simulink model "fft_HIL"  (Simulink 7.0)
settings: Solver=FixedStepDiscrete  StartTime=0.0  StopTime=800  RelTol=1e-3
InitFcn:
  | %% DSPBuilder Start
  | alt_dspbuilder_update_model(bdroot)
  | %% DSPBuilder End
libraries: allblocks_alteradspbuilder2 x18, dspsrcs4 x4, simulink x3
settings Model: Creator=lkong  LastModifiedBy=lkong
settings OptimizationCC: InlineInvariantSignals=on
settings DebuggingCC: SaveWithParameterizedLinksMsg=none  SignalResolutionControl=TryResolveAllWithWarning  SolverPrmCheckMsg=none  MultiTaskDSMMsg=warning  MultiTaskCondExecSysMsg=none
settings HardwareCC: TargetUnknown=on
settings RTWCC: IncludeERTFirstTime=on
settings GRTTargetCC: TargetFcnLib=ansi_tfl_tmw.mat

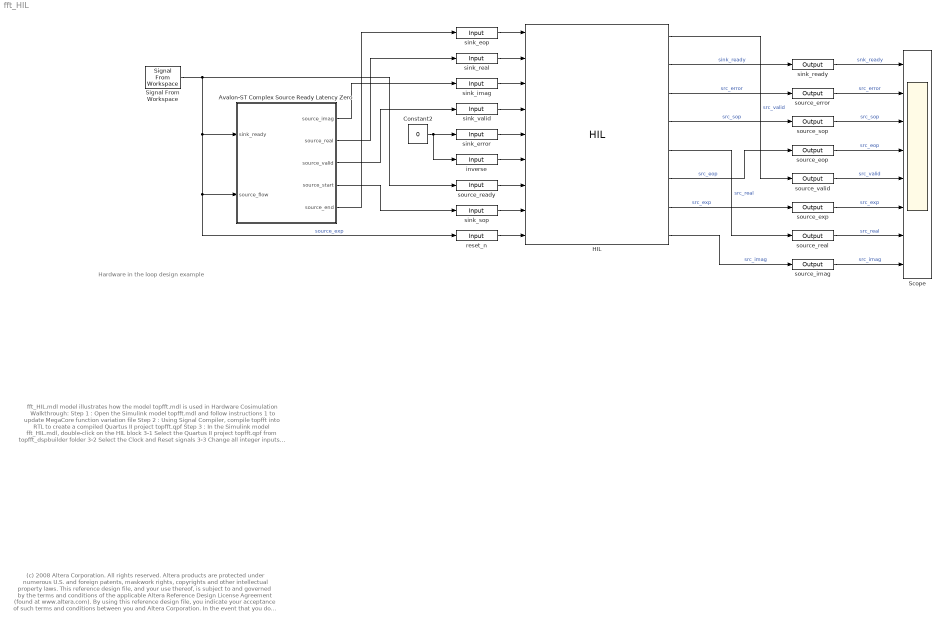
== system fft_HIL ==
  note: (c) 2008 Altera Corporation. All rights reserved.  Altera products are protected under numerous U.S. and foreign patents, maskwork rights, copyrights and other intellectual property laws.
      | This reference design file, and your use thereof, is subject to and governed by the terms and conditions of the applicable Altera Reference Design License Agreement (found at www.altera.com).
      | By using this reference design file, you indicate your acceptance of such terms and conditions between you and Altera Corporation.
      | In the event that you do not agree with such terms and conditions, you may not use the reference design file and please promptly destroy any copies you have made.
      | This reference design file being provided on an "as-is" basis and as an accommodation and therefore all warranties, representations or guarantees of any kind (whether express, implied or statutory)
      | including, without limitation, warranties of merchantability, non-infringement, or fitness for a particular purpose, are specifically disclaimed.
      | By making this reference design file available, Altera expressly does not recommend, suggest or require that this reference design file be used in combination with any other product not provided by Altera
  note: Hardware in the loop design example
  note: fft_HIL.mdl model illustrates how the model topfft.mdl is used in Hardware Cosimulation
      |
      | Walkthrough:
      | Step 1 : Open the Simulink model topfft.mdl and follow instructions 1 to update MegaCore function variation file
      | Step 2 : Using Signal Compiler, compile topfft into RTL to create a compiled Quartus II project topfft.qpf
      | Step 3 : In the Simulink model fft_HIL.mdl, double-click on the HIL block
      |               3-1 Select the Quartus II project topfft.qpf from topfft_dspbuilder folder
      |               3-2 Select the Clock and Reset signals
      |               3-3 Change all integer inputs and outputs to signed
      |               3-4 Select the reset active level to match the settings in the original model
      |               3-5 Click on "Next" to go to page 2 of 2
      |               3-6 Enter the FPGA device value
      |               3-7 Compile with Quartus II
      |               3-8 Select the JTAG cable
      |               3-9 Program the FPGA on board
      |               3-10 Close the HIL dialog box
      | Step 4 : Simulate in Simulink
      |              4-1 Make sure that all inputs to the HIL block are connected up correctly before running simulation
      |              4-2 The FPGA needs to be reprogrammed before running repeated HIL simulation
      |              4-3 If burst mode is used in HIL simulation, extra steps should be added to the Simulation End time
  Avalon-ST Complex Source Ready Latency Zero : Subsystem  mask{datastring=[1:32], sopstring=[1 zeros(1,63)], eopstring=[zeros(1,63) 1], finaloption=Cyclic Repetition}
      mask prompts: datastring "Complex Data"; sopstring "Start of Packet"; eopstring "End of Packet"; finaloption "Form output after final data by"
      mask StyleString: edit,edit,edit,popup(Cyclic Repetition)
      mask Display:
      | port_label('input',1,'sink_ready');
      | port_label('input',2,'source_flow');
      | 
      | port_label('output',1,'source_imag');
      | port_label('output',2,'source_real');
      | port_label('output',3,'source_valid');
      | port_label('output',4,'source_start');
      | port_label('output',5,'source_end');
      | 
      | disp(&1);
  Constant2 : Constant  Value=0  OutDataType=sfix(16)  OutScaling=2^0
  HIL : allblocks_alteradspbuilder2/HIL  entityName=topfft  inNames=sink_eop sink_real sink_imag sink_valid sink_error reset_n inverse source_ready sink_sop  inBwls="1  16  16   1   2   1   1   1   1   1   1"  inBwrs="0  0  0  0  0  0  0  0  0  0  0"  inTypes=b s s b s b b b b  inDelayed="0  0  0  0  0  0  0  0  0"  outNames=source_valid sink_ready source_error source_sop source_real source_eop source_exp source_imag  outBwls="1   1   2   1  16   1   6  16"  outBwrs="0  0  0  0  0  0  0  0"  outTypes=b b s b s b s s  resetNames=aclr  InputCount=11  InputNames=sink_eop sink_real sink_imag Clock sink_valid sink_error reset_n aclr inverse source_ready sink_sop  InputWidth="1  16  16   1   1   2   1   1   1   1   1"  InputRepresentation="0  1  1  0  0  1  0  0  0  0  0"  InputExport="0  0  0  2  0  0  0  3  0  0  0"  InputFPP="0  0  0  0  0  0  0  0  0  0  0"  OutputCount=8  OutputNames=source_valid sink_ready source_error source_sop source_real source_eop source_exp source_imag  OutputWidth="1   1   2   1  16   1   6  16"  OutputRepresentation="0  0  1  0  1  0  1  1"  OutputExport="0  0  0  0  0  0  0  0"  OutputFPP="0  0  0  0  0  0  0  0"  JtagCable=3  JtagDevice=1  BurstMode=off  BurstLength=1024  FrameMode=off  SOP=1  OutValid=1  QuartusProject=D:\P4DspbStd81\p4ws\dsp_builder2\Documentation\DesignExamples\Tutorials\HIL\FFT\topfft_dspbuilder\topfft.qpf  HilNewConfig=off  ClockPinLocation=K17  ClockPinSource=0  HilDeviceOnBoard=EP2S180F1020C5  DR_length=48  dspbuilder_reset=on  SLD_NODE_INFO=4634079  AssertSclrBeforeSimulation=1  SampleTime=-1  dspb_ver=6.1  ResetLevel=Active_High  JtagCableName=USB-Blaster [USB-0]  JtagDeviceName=@1: EP2S180 (0x020960DD)  ClockNames=Clock
  Scope : Scope  NumInputPorts=8
      settings: TimeRange=800  YMin=0~0~-1~-4~-20~-10~0~0  YMax=1~1~1~0~30~70~1~1
  Signal From Workspace : dspsrcs4/Signal From Workspace  SystemSampleTime=-1  X=[0 1]  Ts=1  nsamps=1  OutputAfterFinalValue=Holding final value  ignoreOrWarnInputAndFrameLengths=off
  inverse : allblocks_alteradspbuilder2/Input  iofile=d:\P4DspbStd81\p4ws\dsp_builder2\documentation\designExamples\tutorials\hIL\fFT\tb_fft_HIL\fft%5FHIL_inverse.salt  BusType=Single Bit  bwl=1  bwr=0  SpecifyClock=off  PORTTYPE=Input  externalType=Inferred  allowFloatingPointOverride=on  logOutputs=off
  reset_n : allblocks_alteradspbuilder2/Input  iofile=d:\P4DspbStd81\p4ws\dsp_builder2\documentation\designExamples\tutorials\hIL\fFT\tb_fft_HIL\fft%5FHIL_reset%5Fn.salt  BusType=Single Bit  bwl=1  bwr=0  SpecifyClock=off  PORTTYPE=Input  externalType=Inferred  allowFloatingPointOverride=on  logOutputs=off
  sink_eop : allblocks_alteradspbuilder2/Input  iofile=d:\P4DspbStd81\p4ws\dsp_builder2\documentation\designExamples\tutorials\hIL\fFT\tb_fft_HIL\fft%5FHIL_sink%5Feop.salt  BusType=Single Bit  bwl=1  bwr=0  SpecifyClock=off  PORTTYPE=Input  externalType=Inferred  allowFloatingPointOverride=on  logOutputs=off
  sink_error : allblocks_alteradspbuilder2/Input  iofile=d:\P4DspbStd81\p4ws\dsp_builder2\documentation\designExamples\tutorials\hIL\fFT\tb_fft_HIL\fft%5FHIL_sink%5Ferror.salt  BusType=Signed Integer  bwl=2  bwr=0  SpecifyClock=off  PORTTYPE=Input  externalType=Inferred  allowFloatingPointOverride=on  logOutputs=off
  sink_imag : allblocks_alteradspbuilder2/Input  iofile=d:\P4DspbStd81\p4ws\dsp_builder2\documentation\designExamples\tutorials\hIL\fFT\tb_fft_HIL\fft%5FHIL_sink%5Fimag.salt  BusType=Signed Integer  bwl=16  bwr=0  SpecifyClock=off  PORTTYPE=Input  externalType=Inferred  allowFloatingPointOverride=on  logOutputs=off
  sink_ready : allblocks_alteradspbuilder2/Output  iofile=d:\P4DspbStd81\p4ws\dsp_builder2\documentation\designExamples\tutorials\hIL\fFT\tb_fft_HIL\fft%5FHIL_sink%5Fready.capture  BusType=Single Bit  bwl=1  bwr=0  externalType=Inferred  PORTTYPE=Output  allowFloatingPointOverride=on  logOutputs=off
  sink_real : allblocks_alteradspbuilder2/Input  iofile=d:\P4DspbStd81\p4ws\dsp_builder2\documentation\designExamples\tutorials\hIL\fFT\tb_fft_HIL\fft%5FHIL_sink%5Freal.salt  BusType=Signed Integer  bwl=16  bwr=0  SpecifyClock=off  PORTTYPE=Input  externalType=Inferred  allowFloatingPointOverride=on  logOutputs=off
  sink_sop : allblocks_alteradspbuilder2/Input  iofile=d:\P4DspbStd81\p4ws\dsp_builder2\documentation\designExamples\tutorials\hIL\fFT\tb_fft_HIL\fft%5FHIL_sink%5Fsop.salt  BusType=Single Bit  bwl=1  bwr=0  SpecifyClock=off  PORTTYPE=Input  externalType=Inferred  allowFloatingPointOverride=on  logOutputs=off
  sink_valid : allblocks_alteradspbuilder2/Input  iofile=d:\P4DspbStd81\p4ws\dsp_builder2\documentation\designExamples\tutorials\hIL\fFT\tb_fft_HIL\fft%5FHIL_sink%5Fvalid.salt  BusType=Single Bit  bwl=1  bwr=0  SpecifyClock=off  PORTTYPE=Input  externalType=Inferred  allowFloatingPointOverride=on  logOutputs=off
  source_eop : allblocks_alteradspbuilder2/Output  iofile=d:\P4DspbStd81\p4ws\dsp_builder2\documentation\designExamples\tutorials\hIL\fFT\tb_fft_HIL\fft%5FHIL_source%5Feop.capture  BusType=Single Bit  bwl=1  bwr=0  externalType=Inferred  PORTTYPE=Output  allowFloatingPointOverride=on  logOutputs=off
  source_error : allblocks_alteradspbuilder2/Output  iofile=d:\P4DspbStd81\p4ws\dsp_builder2\documentation\designExamples\tutorials\hIL\fFT\tb_fft_HIL\fft%5FHIL_source%5Ferror.capture  BusType=Signed Integer  bwl=2  bwr=0  externalType=Inferred  PORTTYPE=Output  allowFloatingPointOverride=on  logOutputs=off
  source_exp : allblocks_alteradspbuilder2/Output  iofile=d:\P4DspbStd81\p4ws\dsp_builder2\documentation\designExamples\tutorials\hIL\fFT\tb_fft_HIL\fft%5FHIL_source%5Fexp.capture  BusType=Signed Integer  bwl=6  bwr=0  externalType=Inferred  PORTTYPE=Output  allowFloatingPointOverride=on  logOutputs=off
  source_imag : allblocks_alteradspbuilder2/Output  iofile=d:\P4DspbStd81\p4ws\dsp_builder2\documentation\designExamples\tutorials\hIL\fFT\tb_fft_HIL\fft%5FHIL_source%5Fimag.capture  BusType=Signed Integer  bwl=16  bwr=0  externalType=Inferred  PORTTYPE=Output  allowFloatingPointOverride=on  logOutputs=off
  source_ready : allblocks_alteradspbuilder2/Input  iofile=d:\P4DspbStd81\p4ws\dsp_builder2\documentation\designExamples\tutorials\hIL\fFT\tb_fft_HIL\fft%5FHIL_source%5Fready.salt  BusType=Single Bit  bwl=1  bwr=0  SpecifyClock=off  PORTTYPE=Input  externalType=Inferred  allowFloatingPointOverride=on  logOutputs=off
  source_real : allblocks_alteradspbuilder2/Output  iofile=d:\P4DspbStd81\p4ws\dsp_builder2\documentation\designExamples\tutorials\hIL\fFT\tb_fft_HIL\fft%5FHIL_source%5Freal.capture  BusType=Signed Integer  bwl=16  bwr=0  externalType=Inferred  PORTTYPE=Output  allowFloatingPointOverride=on  logOutputs=off
  source_sop : allblocks_alteradspbuilder2/Output  iofile=d:\P4DspbStd81\p4ws\dsp_builder2\documentation\designExamples\tutorials\hIL\fFT\tb_fft_HIL\fft%5FHIL_source%5Fsop.capture  BusType=Single Bit  bwl=1  bwr=0  externalType=Inferred  PORTTYPE=Output  allowFloatingPointOverride=on  logOutputs=off
  source_valid : allblocks_alteradspbuilder2/Output  iofile=d:\P4DspbStd81\p4ws\dsp_builder2\documentation\designExamples\tutorials\hIL\fFT\tb_fft_HIL\fft%5FHIL_source%5Fvalid.capture  BusType=Single Bit  bwl=1  bwr=0  externalType=Inferred  PORTTYPE=Output  allowFloatingPointOverride=on  logOutputs=off
  wires:
  Avalon-ST Complex Source Ready Latency Zero/3(source_valid) -> sink_valid/1
  Avalon-ST Complex Source Ready Latency Zero/5(source_end) -> sink_eop/1
  Signal From Workspace/1 -> Avalon-ST Complex Source Ready Latency Zero/2(source_flow), reset_n/1, Avalon-ST Complex Source Ready Latency Zero/1(sink_ready), source_ready/1  "source_exp"
  Constant2/1 -> sink_error/1, inverse/1
  Avalon-ST Complex Source Ready Latency Zero/1(source_imag) -> sink_imag/1
  Avalon-ST Complex Source Ready Latency Zero/2(source_real) -> sink_real/1
  sink_imag/1 -> HIL/3
  sink_real/1 -> HIL/2
  sink_error/1 -> HIL/5
  sink_eop/1 -> HIL/1
  sink_valid/1 -> HIL/4
  inverse/1 -> HIL/6
  source_ready/1 -> HIL/7
  sink_sop/1 -> HIL/8
  reset_n/1 -> HIL/9
  Avalon-ST Complex Source Ready Latency Zero/4(source_start) -> sink_sop/1
  HIL/2 -> sink_ready/1  "sink_ready"
  HIL/3 -> source_error/1  "src_error"
  HIL/1 -> source_valid/1  "src_valid"
  HIL/5 -> source_real/1  "src_real"
  source_eop/1 -> Scope/4  "src_eop"
  source_error/1 -> Scope/2  "src_error"
  source_exp/1 -> Scope/6  "src_exp"
  source_imag/1 -> Scope/8  "src_imag"
  source_real/1 -> Scope/7  "src_real"
  source_sop/1 -> Scope/3  "src_sop"
  source_valid/1 -> Scope/5  "src_valid"
  sink_ready/1 -> Scope/1  "snk_ready"
  HIL/4 -> source_sop/1  "src_sop"
  HIL/6 -> source_eop/1  "src_eop"
  HIL/7 -> source_exp/1  "src_exp"
  HIL/8 -> source_imag/1  "src_imag"

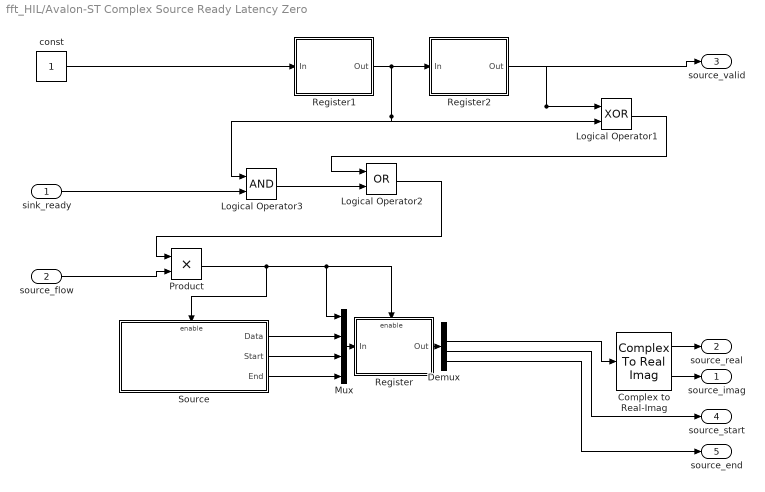
== system fft_HIL/Avalon-ST Complex Source Ready Latency Zero ==
  sink_ready : Inport  OutDataType=sfix(16)  OutScaling=2^0
  source_flow : Inport  Port=2  OutDataType=sfix(16)  OutScaling=2^0
  Complex to Real-Imag : ComplexToRealImag
  Demux : Demux
  Logical Operator1 : Logic  Operator=XOR  AllPortsSameDT=off  OutDataTypeMode=boolean
  Logical Operator2 : Logic  Operator=OR  AllPortsSameDT=off  OutDataTypeMode=boolean
  Logical Operator3 : Logic  AllPortsSameDT=off  OutDataTypeMode=boolean
  Mux : Mux
  Product : Product  OutDataType=sfix(16)  OutScaling=2^0  RndMeth=Zero
  Register : Subsystem  TreatAsAtomicUnit=on
  Register1 : Subsystem  TreatAsAtomicUnit=on
  Register2 : Subsystem  TreatAsAtomicUnit=on
  Source : Subsystem  TreatAsAtomicUnit=on  mask{datastring=datastring, sopstring=sopstring, eopstring=eopstring}
      mask prompts: datastring "Complex Data"; sopstring "Start of Packet"; eopstring "End of Packet"
  const : Constant  OutDataType=sfix(16)  OutScaling=2^0
  source_imag : Outport  OutDataType=sfix(16)  OutScaling=2^0
  source_real : Outport  Port=2  OutDataType=sfix(16)  OutScaling=2^0
  source_valid : Outport  Port=3  OutDataType=sfix(16)  OutScaling=2^0
  source_start : Outport  Port=4  OutDataType=sfix(16)  OutScaling=2^0
  source_end : Outport  Port=5  OutDataType=sfix(16)  OutScaling=2^0
  wires:
  Demux/4 -> source_end/1
  Demux/3 -> source_start/1
  Demux/2 -> Complex to Real-Imag/1
  Source/1(Data) -> Mux/2
  Source/2(Start) -> Mux/3
  Source/3(End) -> Mux/4
  Complex to Real-Imag/2 -> source_imag/1
  Complex to Real-Imag/1 -> source_real/1
  Register/1(Out) -> Demux/1
  Mux/1 -> Register/1(In)
  Product/1 -> Source/Enable, Mux/1, Register/Enable
  source_flow/1 -> Product/2
  Register1/1(Out) -> Register2/1(In), Logical Operator1/2, Logical Operator3/1
  const/1 -> Register1/1(In)
  Register2/1(Out) -> Logical Operator1/1, source_valid/1
  sink_ready/1 -> Logical Operator3/2
  Logical Operator1/1 -> Logical Operator2/1
  Logical Operator2/1 -> Product/1
  Logical Operator3/1 -> Logical Operator2/2

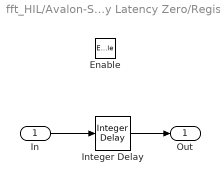
== system fft_HIL/Avalon-ST Complex Source Ready Latency Zero/Register ==
  In : Inport  OutDataType=sfix(16)  OutScaling=2^0
  Enable : EnablePort
  Integer Delay : simulink/Discrete/Integer Delay  vinit=0.0  samptime=-1  NumDelays=1
  Out : Outport  OutDataType=sfix(16)  OutScaling=2^0
  wires:
  Integer Delay/1 -> Out/1
  In/1 -> Integer Delay/1

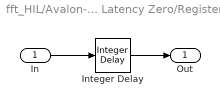
== system fft_HIL/Avalon-ST Complex Source Ready Latency Zero/Register1 ==
  In : Inport  OutDataType=sfix(16)  OutScaling=2^0
  Integer Delay : simulink/Discrete/Integer Delay  vinit=0.0  samptime=-1  NumDelays=1
  Out : Outport  OutDataType=sfix(16)  OutScaling=2^0
  wires:
  Integer Delay/1 -> Out/1
  In/1 -> Integer Delay/1

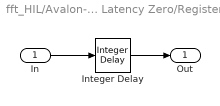
== system fft_HIL/Avalon-ST Complex Source Ready Latency Zero/Register2 ==
  In : Inport  OutDataType=sfix(16)  OutScaling=2^0
  Integer Delay : simulink/Discrete/Integer Delay  vinit=0.0  samptime=-1  NumDelays=1
  Out : Outport  OutDataType=sfix(16)  OutScaling=2^0
  wires:
  Integer Delay/1 -> Out/1
  In/1 -> Integer Delay/1

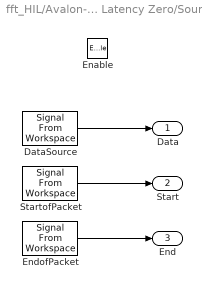
== system fft_HIL/Avalon-ST Complex Source Ready Latency Zero/Source ==
  Enable : EnablePort
  DataSource : dspsrcs4/Signal From Workspace  X=datastring  Ts=-1  nsamps=1  OutputAfterFinalValue=Cyclic repetition  ignoreOrWarnInputAndFrameLengths=off
  EndofPacket : dspsrcs4/Signal From Workspace  X=eopstring  Ts=-1  nsamps=1  OutputAfterFinalValue=Cyclic repetition  ignoreOrWarnInputAndFrameLengths=off
  StartofPacket : dspsrcs4/Signal From Workspace  X=sopstring  Ts=-1  nsamps=1  OutputAfterFinalValue=Cyclic repetition  ignoreOrWarnInputAndFrameLengths=off
  Data : Outport  OutDataType=sfix(16)  OutScaling=2^0
  Start : Outport  Port=2  OutDataType=sfix(16)  OutScaling=2^0
  End : Outport  Port=3  OutDataType=sfix(16)  OutScaling=2^0
  wires:
  EndofPacket/1 -> End/1
  StartofPacket/1 -> Start/1
  DataSource/1 -> Data/1
